simulink model "practica_5"  (R2024b)
settings: Solver=VariableStepAuto  StartTime=0.0  StopTime=0.25  RelTol=1e-6
undefined symbols (not defined in the file): den, num
settings Model: Creator=diegp  LastModifiedBy=diegp

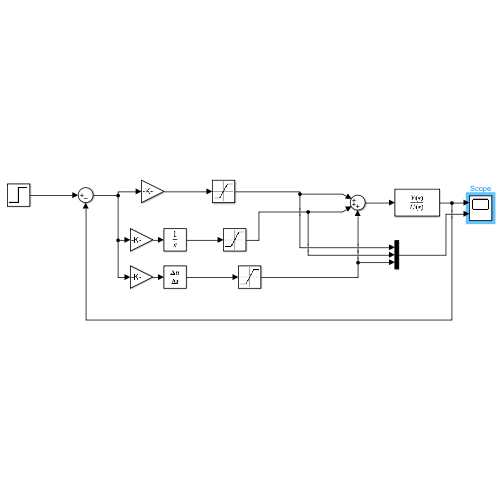
[thumbnail: Simulink's stored preview of the top-level diagram]
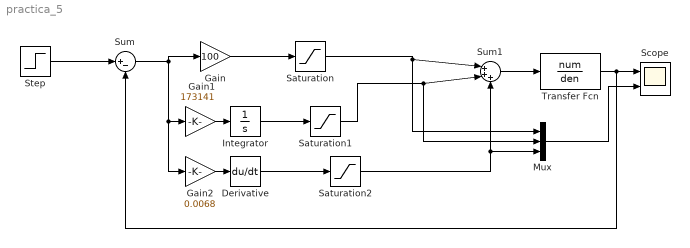
== system practica_5 ==
  Derivative : Derivative
  Gain : Gain  Gain=100
  Gain1 : Gain  Gain=173141
  Gain2 : Gain  Gain=0.0068
  Integrator : Integrator
  Mux : Mux  Inputs=3
  Saturation : Saturate  UpperLimit=15  LowerLimit=-15
  Saturation1 : Saturate  UpperLimit=15  LowerLimit=-15
  Saturation2 : Saturate  UpperLimit=15  LowerLimit=-15
  Scope : Scope  NumInputPorts=2
  Step : Step  Time=0.01  SampleTime=0
  Sum : Sum  Inputs=|+-
  Sum1 : Sum  Inputs=|+++
  Transfer Fcn : TransferFcn  Numerator=num  Denominator=den
  wires:
  Transfer Fcn/1 -> Sum/2, Scope/1
  Step/1 -> Sum/1
  Sum/1 -> Gain2/1, Gain1/1, Gain/1
  Gain1/1 -> Integrator/1
  Gain/1 -> Saturation/1
  Integrator/1 -> Saturation1/1
  Sum1/1 -> Transfer Fcn/1
  Gain2/1 -> Derivative/1
  Derivative/1 -> Saturation2/1
  Saturation/1 -> Mux/1, Sum1/1
  Saturation1/1 -> Mux/2, Sum1/2
  Saturation2/1 -> Mux/3, Sum1/3
  Mux/1 -> Scope/2
